simulink model "Controller_HIL"  (R2023b)
settings: Solver=FixedStepDiscrete  StartTime=0.0  StopTime=inf  FixedStep=ts_controller  RelTol=1e-3
InitFcn:
  | mbd_s32k_consistency_checks(bdroot(gcs));
undefined symbols (not defined in the file): Battery, BMS_Controller_State, Charging_State, currentFactor, CV_Gain, DiscIntNeverNeededParam, I_cc, LQFP, MaxCellVoltThrsld, noCurrent, Ns_Module, NumModules, OverCellVoltageLimit, SOCInit, SRE, ts_controller, ts_system, UnderCellVoltageLimit, voltThreshold
libraries: mbd_s32k1xx_ec_toolbox x20, mbd_bcc_ec_toolbox x16, etargetslib x11, simulink x5, sharedTrackingLibrary x2, hdlsllib x1
(part 1 of 2)
settings Model: DataDictionary=System.sldd  EnableAccessToBaseWorkspace=off  Creator=vasileios.amoiridis  LastModifiedBy=jatin.anand
settings DataIOCC: ExternalInput=off  InitialState=off  SaveOutput=off  SignalLogging=off  SaveTime=off
settings OptimizationCC: DefaultParameterBehavior=Inlined  DefaultUnderspecifiedDataType=single  EnhancedBackFolding=on  PassReuseOutputArgsAs=Individual arguments  ZeroExternalMemoryAtStartup=off  ZeroInternalMemoryAtStartup=off  OptimizeBlockOrder=speed  DifferentSizesBufferReuse=on  OptimizationCustomize=off  EfficientTunableParamExpr=on
settings DebuggingCC: InheritedTsInSrcMsg=none  SingleTaskRateTransMsg=error  ParameterTunabilityLossMsg=error  UnconnectedInputMsg=error  UnconnectedOutputMsg=error  UnconnectedLineMsg=error  UnknownTsInhSupMsg=error
settings HardwareCC: ProdBitPerPointer=32  ProdBitPerSizeT=32  ProdBitPerPtrDiffT=32  ProdLargestAtomicInteger=Long  ProdLargestAtomicFloat=Double  ProdWordSize=32  ProdHWDeviceType=ARM Compatible->ARM Cortex
settings SFSimCC: MATLABDynamicMemAlloc=off
settings RTWCC: Description=Model Based Design Toolbox S32K1xx Code Generation Target  SystemTargetFile=mbd_s32k.tlc  MakeCommand=mbd_s32k_make_rtw COPY_MDLREF_INCLUDES=0  TemplateMakefile=mbd_s32k.tmf
settings CodeAppCC: ForceParamTrailComments=on  IgnoreCustomStorageClasses=off  OperatorAnnotations=on  SimulinkDataObjDesc=on  SFDataObjDesc=on  InsertBlockDesc=on
settings STFCustomTargetCC: MultiwordLength=256  CombineOutputUpdateFcns=on  ERTCustomFileBanners=on  SupportContinuousTime=off  SupportNonInlinedSFcns=off  RemoveResetFunc=on  MATLABClassNameForMDSCustomization=Simulink.SoftwareTarget.ERTCustomization  SystemTargetFile=mbd_s32k.tlc
settings ERTTargetCC: TargetLangStandard=C99 (ISO)  ParMdlRefBuildCompliant=off  CompOptLevelCompliant=off  ConcurrentExecutionCompliant=off  ModelStepFunctionPrototypeControlCompliant=off  CPPClassGenCompliant=off  UseToolchainInfoCompliant=off  InlinedParameterPlacement=NonHierarchical  ERTSrcFileBannerTemplate=mbd_ert_code_template.cgt  ERTHdrFileBannerTemplate=mbd_ert_code_template.cgt  ERTDataSrcFileTemplate=mbd_ert_code_template.cgt  ERTDataHdrFileTemplate=mbd_ert_code_template.cgt  ERTCustomFileTemplate=example_file_process.tlc

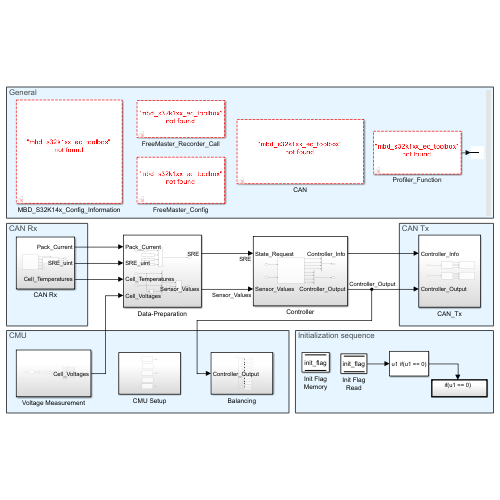
[thumbnail: Simulink's stored preview of the top-level diagram]
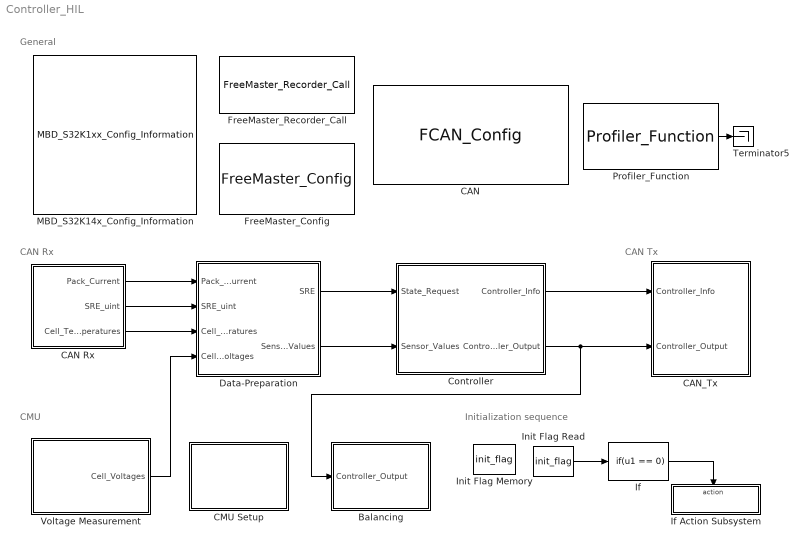
== system Controller_HIL ==
  note: CAN Tx
  note: CAN Rx
  note: CMU
  note: General
  note: Initialization sequence
  Balancing : Subsystem
  CAN : mbd_s32k1xx_ec_toolbox/Communication Blocks/CAN Blocks/FCAN_Config  Priority=1  can_instance=0  can_mode=Normal mode  can_max_num_mb=32  can_rx=PTE4: [CAN0_RX | CAN Rx channel]  can_tx=PTE5: [CAN0_TX | CAN Tx Channel]  show_adv_opts=on  can_clk_src=Peripheral clock  can_clk_freq=80 MHz  bitrate_to_time_seg=on  bitrate=1000  sample_point=80  real_bitrate=1000  real_sample_point=80  prop_delay=250  bus_length=1  tq=100.0  time_quanta=10  can_presdiv=8  can_propseg=6  can_pseg1=1  can_pseg2=2  can_rjw=1  cbt_bitrate=2000  cbt_sample_point=87.5  cbt_real_bitrate=2000  cbt_real_sample_point=80  cbt_tq=12.5  cbt_time_quanta=40  can_cbt_presdiv=1  can_cbt_propseg=29  can_cbt_pseg1=5  can_cbt_pseg2=5  can_cbt_rjw=5  can_fd_enable=off  can_payload=8  tdc_enable=off  tdc_offset=20  can_rxfifo_enable=on  can_num_id_filters=16  can_fifo_id_format=A  can_fifo_id_filter={{false,false,'0x401'},{false,false,'0x402'},{false,false,'0x403'},{false,false,'0x404'},{false,false,'0x405'},{false,false,'0x406'},{false,false,'0x407'},{false,false,'0x408'},{false,false,'0x409'},{false,false,'0x0'},{false,false,'0x0'},{false,false,'0x0'},{false,false,'0x0'},{false,false,'0x0'},{false,false,'0x0'},{false,false,'0x0'}}  can_pn_enable=off  can_wakeup_match=off  can_wakeup_timeout=off  can_timeout_en=off  can_match_timeout=1  can_multiple_matches_en=off  can_num_matches=1  can_idfilter_extendedid=off  can_idfilter_remoteframe=off  can_idfilter_type=Match exact  can_idfilter_id1=0  can_idfilter_id2=0  can_payloadfilter_enable=off  can_payloadfilter_dlclow=0  can_payloadfilter_dlchigh=0  can_payloadfilter_type=Match exact  can_payloadfilter_payload1_b0=0  can_payloadfilter_payload1_b1=0  can_payloadfilter_payload1_b2=0  can_payloadfilter_payload1_b3=0  can_payloadfilter_payload1_b4=0  can_payloadfilter_payload1_b5=0  can_payloadfilter_payload1_b6=0  can_payloadfilter_payload1_b7=0  can_payloadfilter_payload2_b0=0  can_payloadfilter_payload2_b1=0  can_payloadfilter_payload2_b2=0  can_payloadfilter_payload2_b3=0  can_payloadfilter_payload2_b4=0  can_payloadfilter_payload2_b5=0  can_payloadfilter_payload2_b6=0  can_payloadfilter_payload2_b7=0
  CAN Rx : Subsystem
  CAN_Tx : Subsystem
  CMU Setup : Subsystem
  Controller : Subsystem
  Data-Preparation : Subsystem
  FreeMaster_Config : mbd_s32k1xx_ec_toolbox/Utility Blocks/FreeMaster_Config  interface=LPUART1  baudrate=115200  rxd=PTC6: [LPUART1_RX | Receive]  txd=PTC7: [LPUART1_TX | Transmit]  mode=Short Interrupt  isr_prio=1  show_adv_opts=on  use_scope=on  max_scope_vars=8  use_recorder=on  max_rec_vars=8  rec_buff_size=512  rec_timebase=100 milliseconds  comm_buffer_size_auto=on  comm_buffer_size=255  comm_rqueue_size_default=on  comm_rqueue_size=32
  FreeMaster_Recorder_Call : mbd_s32k1xx_ec_toolbox/Utility Blocks/FreeMaster_Recorder_Call
  If : If  IfExpression=u1 == 0  ShowElse=off
  If Action Subsystem : Subsystem  TreatAsAtomicUnit=on
  Init Flag Memory : DataStoreMemory  DataStoreName=init_flag  ReadBeforeWriteMsg=warning  WriteAfterWriteMsg=warning  WriteAfterReadMsg=warning  ShowAdditionalParam=off  OutDataTypeStr=uint32
  Init Flag Read : DataStoreRead  DataStoreName=init_flag  IndexOptions=Index vector (dialog)  Indices=1  OutputSizes=1
  MBD_S32K14x_Config_Information : mbd_s32k1xx_ec_toolbox/MBD_S32K1xx_Config_Information  Priority=0  mbdt_ver=0  disp_str=|  config_params=[]  mcu_target_name=S32K144  mcu_target_package=100-LQFP  mcu_target_sram_size=48KB  mcu_system_clock_freq=80  mcu_xtal_freq=External 8  mcu_steptick_timer=LPIT Channel 0  mcu_steptick_prio=3  ds_import_enable=on  target_compiler=GCC  target_memory=FLASH  gcc_target_compile_opts=-mthumb -mfloat-abi=hard -mfpu=fpv4-sp-d16 -O1 -g -gstrict-dwarf  gcc_target_assemble_opts=-mthumb -mfloat-abi=hard -mfpu=fpv4-sp-d16 -g  gcc_target_link_opts=-mthumb -mfloat-abi=hard -mfpu=fpv4-sp-d16  gcc_target_default_lcf=on  gcc_target_user_lcf=S32K144_48_flash.ld  ghs_target_compile_opts=-cpu=cortexm4f -thumb -DARM_MATH_CM4 -fpu=vfpv4_d16 -fsingle -Ogeneral -Wundef -Wimplicit-int -Wshadow -Wtrigraphs --no_commons --gnu_asm -gnu99 -gdwarf-2 -G  ghs_target_assemble_opts=-cpu=cortexm4f -fpu=vfpv4_d16  ghs_target_link_opts=-cpu=cortexm4f -thumb -fpu=vfpv4_d16  ghs_target_default_lcf=off  ghs_target_user_lcf=S32K144_48_flash.ld  iar_target_compile_opts=--cpu=Cortex-M4F --thumb --fpu=VFPv4_sp -Ol -e --debug --dlib_config normal  iar_target_assemble_opts=--cpu Cortex-M4F --thumb --fpu VFPv4_sp  iar_target_link_opts=--no_exceptions --vfe --inline  iar_target_default_lcf=off  iar_target_user_lcf=S32K144_48_flash.icf  pil_download_enable=off  rbl_download_enable=on  rbl_start_delay=5000000  rbl_download_interface=OpenSDA  rbl_restart_request=off  rbl_com_port=Custom  rbl_com_port_custom=COM1  pil_download_rate=57600  pil_download_rate_custom=115200  pil_opensda_drive=Custom  pil_opensda_drive_custom=D  jtag_interface=OpenSDA Embedded Debug  jlink_default_path=on  jlink_user_path=C:\Program Files\SEGGER\JLink\  pil_uart_instance=1  pil_uart_rx=PTC6: [LPUART1_RX | Receive]  pil_uart_tx=PTC7: [LPUART1_TX | Transmit]  FTM_PWM_PcrCheckEnDis=on  FTM_Input_Edge_Inputs_PcrCheckEnDis=on  FTM_Dual_Edge_Inputs_PcrCheckEnDis=on  FTM_Quadrature_Inputs_PcrCheckEnDis=on  FTM_Hall_Sensor_Inputs_PcrCheckEnDis=on  LPTMR_PcrCheckEnDis=on  PIT_PcrCheckEnDis=on  RTC_PcrCheckEnDis=on  FlexCAN_PcrCheckEnDis=on  LIN_PcrCheckEnDis=on  FlexIO_PcrCheckEnDis=on  LPI2C_PcrCheckEnDis=on  LPSPI_PcrCheckEnDis=on  LPUART_PcrCheckEnDis=on  CMP_PcrCheckEnDis=on  GPIO_OutputPcrCheckEnDis=on  GPIO_InputPcrCheckEnDis=on  SBC_PcrCheckEnDis=on  BMS_PcrCheckEnDis=on  AMMCLIB_PcrCheckEnDis=on  FM_PcrCheckEnDis=on  Profile_PcrCheckEnDis=on  ConfigParams_PcrCheckEnDis=on  ModelRef_PcrCheckEnDis=on  PDB0_PcrCheckEnDis=on  CSEc_PcrCheckEnDis=on  eDMA_PcrCheckEnDis=on  FLASH_PcrCheckEnDis=on  ADC_PcrCheckEnDis=on  WDOG_PcrCheckEnDis=on
      | Target : S32K144-64KB_SRAM
      | Package : 100-pin
      | System clock : 80 MHz
      | XTAL clock : External 8 MHz
      | Compiler : GCC
      | Target Type : FLASH
      | Download Code after build : (OpenSDA: E)
      | Step Tick Interrupt Priority : 15
  Profiler_Function : mbd_s32k1xx_ec_toolbox/Utility Blocks/Profiler_Function  profile_indx=0
      settings: showOut=on
  Terminator5 : Terminator
  Voltage Measurement : Subsystem
  wires:
  Controller/2(Controller_Output) -> Balancing/1(Controller_Output), CAN_Tx/2(Controller_Output)
  Profiler_Function/1 -> Terminator5/1
  Data-Preparation/2(Sensor_Values) -> Controller/2(Sensor_Values)
  Controller/1(Controller_Info) -> CAN_Tx/1(Controller_Info)
  If/1 -> If Action Subsystem/Action
  Data-Preparation/1(SRE) -> Controller/1(State_Request)
  Init Flag Read/1 -> If/1
  CAN Rx/1(Pack_Current) -> Data-Preparation/1(Pack_Current)
  CAN Rx/2(SRE_uint) -> Data-Preparation/2(SRE_uint)
  CAN Rx/3(Cell_Temperatures) -> Data-Preparation/3(Cell_Temperatures)
  Voltage Measurement/1(Cell_Voltages) -> Data-Preparation/4(Cell_Voltages)

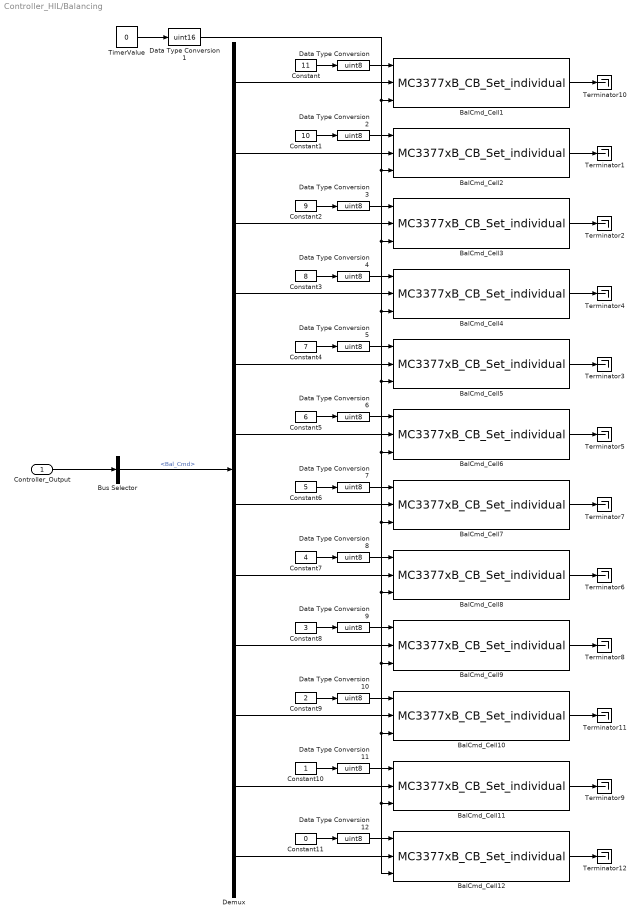
== system Controller_HIL/Balancing ==
  Controller_Output : Inport
  BalCmd_Cell{1..12} (12 alike) : mbd_bcc_ec_toolbox/BMS/MC3377xB_CB_Set_individual  bccInstance=0  bccCID=1
  Bus Selector : BusSelector  OutputSignals=Bal_Cmd
  Constant : Constant  Value=11  SampleTime=-1
  Constant1 : Constant  Value=10  SampleTime=-1
  Constant10 : Constant  SampleTime=-1
  Constant11 : Constant  Value=0  SampleTime=-1
  Constant2 : Constant  Value=9  SampleTime=-1
  Constant3 : Constant  Value=8  SampleTime=-1
  Constant4 : Constant  Value=7  SampleTime=-1
  Constant5 : Constant  Value=6  SampleTime=-1
  Constant6 : Constant  Value=5  SampleTime=-1
  Constant7 : Constant  Value=4  SampleTime=-1
  Constant8 : Constant  Value=3  SampleTime=-1
  Constant9 : Constant  Value=2  SampleTime=-1
  Data Type Conversion{,2..12} (12 alike) : DataTypeConversion  OutDataTypeStr=uint8  SaturateOnIntegerOverflow=off  RndMeth=Floor
  Data Type Conversion1 : DataTypeConversion  OutDataTypeStr=uint16  SaturateOnIntegerOverflow=off  RndMeth=Floor
  Demux : Demux  Outputs=12
  Terminator{1..12} (12 alike) : Terminator
  TimerValue : Constant  Value=0  SampleTime=-1
  wires:
  Demux/12 -> BalCmd_Cell12/2
  Demux/3 -> BalCmd_Cell3/2
  BalCmd_Cell6/1 -> Terminator5/1
  Constant10/1 -> Data Type Conversion11/1
  Demux/10 -> BalCmd_Cell10/2
  BalCmd_Cell10/1 -> Terminator11/1
  Data Type Conversion6/1 -> BalCmd_Cell6/1
  Demux/1 -> BalCmd_Cell1/2
  Demux/5 -> BalCmd_Cell5/2
  Constant8/1 -> Data Type Conversion9/1
  Constant11/1 -> Data Type Conversion12/1
  TimerValue/1 -> Data Type Conversion1/1
  Constant6/1 -> Data Type Conversion7/1
  Data Type Conversion8/1 -> BalCmd_Cell8/1
  Data Type Conversion9/1 -> BalCmd_Cell9/1
  Data Type Conversion5/1 -> BalCmd_Cell5/1
  Constant9/1 -> Data Type Conversion10/1
  Bus Selector/1 -> Demux/1  "<Bal_Cmd>"
  Demux/11 -> BalCmd_Cell11/2
  Data Type Conversion1/1 -> BalCmd_Cell5/3, BalCmd_Cell11/3, BalCmd_Cell12/3, BalCmd_Cell10/3, BalCmd_Cell9/3, BalCmd_Cell8/3, BalCmd_Cell7/3, BalCmd_Cell6/3, BalCmd_Cell4/3, BalCmd_Cell3/3, BalCmd_Cell2/3, BalCmd_Cell1/3
  Demux/9 -> BalCmd_Cell9/2
  BalCmd_Cell7/1 -> Terminator7/1
  Demux/8 -> BalCmd_Cell8/2
  Demux/2 -> BalCmd_Cell2/2
  Demux/7 -> BalCmd_Cell7/2
  Data Type Conversion11/1 -> BalCmd_Cell11/1
  Constant7/1 -> Data Type Conversion8/1
  Constant/1 -> Data Type Conversion/1
  BalCmd_Cell12/1 -> Terminator12/1
  Data Type Conversion7/1 -> BalCmd_Cell7/1
  Data Type Conversion10/1 -> BalCmd_Cell10/1
  BalCmd_Cell5/1 -> Terminator3/1
  BalCmd_Cell8/1 -> Terminator6/1
  Demux/4 -> BalCmd_Cell4/2
  Demux/6 -> BalCmd_Cell6/2
  BalCmd_Cell3/1 -> Terminator2/1
  Controller_Output/1 -> Bus Selector/1
  Data Type Conversion12/1 -> BalCmd_Cell12/1
  Constant3/1 -> Data Type Conversion4/1
  Constant1/1 -> Data Type Conversion2/1
  BalCmd_Cell1/1 -> Terminator10/1
  BalCmd_Cell2/1 -> Terminator1/1
  Constant2/1 -> Data Type Conversion3/1
  Data Type Conversion/1 -> BalCmd_Cell1/1
  BalCmd_Cell4/1 -> Terminator4/1
  BalCmd_Cell9/1 -> Terminator8/1
  Constant5/1 -> Data Type Conversion6/1
  Data Type Conversion3/1 -> BalCmd_Cell3/1
  Data Type Conversion2/1 -> BalCmd_Cell2/1
  Data Type Conversion4/1 -> BalCmd_Cell4/1
  BalCmd_Cell11/1 -> Terminator9/1
  Constant4/1 -> Data Type Conversion5/1

== system Controller_HIL/CAN Rx ==
  FCAN_Rx_FIFO_Complete_Isr : mbd_s32k1xx_ec_toolbox/Communication Blocks/CAN Blocks/FCAN_Isr  can_instance=0  can_event=Rx FIFO Complete
  RX_FIFO_Complete_Event : Subsystem
  Terminator : Terminator
  Terminator1 : Terminator
  Pack_Current : Outport
  SRE_uint : Outport  Port=2
  Cell_Temperatures : Outport  Port=3
  wires:
  FCAN_Rx_FIFO_Complete_Isr/4 -> Terminator/1
  FCAN_Rx_FIFO_Complete_Isr/5 -> Terminator1/1
  FCAN_Rx_FIFO_Complete_Isr/2 -> RX_FIFO_Complete_Event/1(ID)
  FCAN_Rx_FIFO_Complete_Isr/3 -> RX_FIFO_Complete_Event/2(Data)
  FCAN_Rx_FIFO_Complete_Isr/1 -> RX_FIFO_Complete_Event/Trigger
  RX_FIFO_Complete_Event/1(Pack_Current) -> Pack_Current/1
  RX_FIFO_Complete_Event/2(SRE_uint) -> SRE_uint/1
  RX_FIFO_Complete_Event/3(Cell_Temperatures) -> Cell_Temperatures/1

== system Controller_HIL/CAN_Tx ==
  Controller_Info : Inport
  Controller_Output : Inport  Port=2
  CAN_Data : Subsystem
  CAN_Data_HIL : Subsystem
  TX_Complete_HIL : Subsystem  TreatAsAtomicUnit=on
  Tx_Complete : Subsystem  TreatAsAtomicUnit=on
  wires:
  CAN_Data/4(Length_0x202) -> Tx_Complete/4(Length_0x202)
  CAN_Data/3(Data_0x202) -> Tx_Complete/3(Data_0x202)
  CAN_Data/1(Data_0x201) -> Tx_Complete/1(Data_0x201)
  CAN_Data/2(Length_0x201) -> Tx_Complete/2(Length_0x201)
  CAN_Data_HIL/1(Data_0x501) -> TX_Complete_HIL/1(Data_0x501)
  CAN_Data_HIL/2(Length_0x501) -> TX_Complete_HIL/2(Length_0x501)
  CAN_Data_HIL/4(Length_0x502) -> TX_Complete_HIL/4(Length_0x502)
  CAN_Data_HIL/3(Data_0x502) -> TX_Complete_HIL/3(Data_0x502)
  Controller_Info/1 -> CAN_Data_HIL/1(Controller_Info)
  Controller_Output/1 -> CAN_Data/1(Controller_Output)

== system Controller_HIL/CMU Setup ==
  "LPSPI_RX " : mbd_s32k1xx_ec_toolbox/Communication Blocks/SPI Blocks/LPSPI_Config   InstanceNumber=0  Role=Slave  BaudRate=1000000  ShowAdvanced=on  sin=PTB3: [LPSPI0_SIN | LPSPI Serial Data Input]  sout=None  sck=PTB2: [LPSPI0_SCK | LPSPI Serial Clock I/O]  pcs0=None  pcs1=PTB5: [LPSPI0_PCS1 | Peripheral Chip Select 1]  pcs2=None  pcs3=None  CPHA=1  CPOL=0  BitOrder=MSB first  TransferSize=40  WhichPCS=1  PCSPol=ActiveLow  ContinuousTransfer=off
  LPSPI_TX : mbd_s32k1xx_ec_toolbox/Communication Blocks/SPI Blocks/LPSPI_Config   InstanceNumber=1  Role=Master  BaudRate=2000000  ShowAdvanced=on  sin=None  sout=PTB16: [LPSPI1_SOUT | LPSPI Serial Data Output]  sck=PTB14: [LPSPI1_SCK | LPSPI Serial Clock I/O]  pcs0=PTD3: [LPSPI1_PCS0 | Peripheral Chip Select 0]  pcs1=PTA6: [LPSPI1_PCS1 | Peripheral Chip Select 1]  pcs2=None  pcs3=None  CPHA=1  CPOL=0  BitOrder=MSB first  TransferSize=40  WhichPCS=1  PCSPol=ActiveLow  ContinuousTransfer=off
  MC3377xB_CB_Disable_Enable : mbd_bcc_ec_toolbox/BMS/MC3377xB_CB_Disable_Enable  bccInstance=0  bccCID=1  bccAction=Enable
  MC3377xB_Config : mbd_bcc_ec_toolbox/BMS/MC3377xB_Config  Priority=1  bccInstance=0  bccMode=TPL  bccTPLDevNr=1  bccSpiDev=MC33771B  bccSpiCell=3  bccTPLDev1=MC33771B  bccTPLCell1=14  bccTPLDev2=MC33771B  bccTPLCell2=3  bccTPLDev3=MC33771B  bccTPLCell3=3  bccTPLDev4=MC33771B  bccTPLCell4=3  bccTPLDev5=MC33771B  bccTPLCell5=3  bccTPLDev6=MC33771B  bccTPLCell6=3  bccTPLDev7=MC33771B  bccTPLCell7=3  bccTPLDev8=MC33771B  bccTPLCell8=3  bccTPLDev9=MC33771B  bccTPLCell9=3  bccTPLDev10=MC33771B  bccTPLCell10=3  bccTPLDev11=MC33771B  bccTPLCell11=3  bccTPLDev12=MC33771B  bccTPLCell12=3  bccTPLDev13=MC33771B  bccTPLCell13=3  bccTPLDev14=MC33771B  bccTPLCell14=3  bccTPLDev15=MC33771B  bccTPLCell15=3  bccSpiMaster=1  bccSPIMasterCSCustom=off  bccSPIMasterPCS=LPSPI_PCS1  bccSPIMasterPCSGPIO=PTA0: [PTA0 | Port A I/O]  bccSpiSlave=0  bccSPISlavePCS=LPSPI_PCS1  bccSPI_RESET_ALT0=PTA0: [PTA0 | Port A I/O]  bccTPL_ENABLE=PTB0: [PTB0 | Port B I/O]  bccTPL_INTB=PTB1: [PTB1 | Port B I/O]  bccNTCBeta=3900  bccNTCRes=6800  bccNTCRefR=10000  bccNTCRefT=25  bccShunt=10000
  MC3377xB_Start_Conversion : mbd_bcc_ec_toolbox/BMS/MC3377xB_Start_Conversion  Priority=100  bccInstance=0  bccCID=1  bccCIDGlobal=on  bccADCCFG=0
  Terminator : Terminator
  Terminator1 : Terminator
  Terminator2 : Terminator
  wires:
  MC3377xB_CB_Disable_Enable/1 -> Terminator/1
  MC3377xB_Config/1 -> Terminator2/1
  MC3377xB_Start_Conversion/1 -> Terminator1/1

== system Controller_HIL/Controller ==
  State_Request : Inport  OutDataTypeStr=Enum: SRE  PortDimensions=1
  Sensor_Values : Inport  Port=2  OutDataTypeStr=Bus: Sensor_Values  BusOutputAsStruct=on
  Bus Creator : BusCreator  Inputs=4  OutDataTypeStr=Bus: Controller_Info
  Bus Creator1 : BusCreator  Inputs=4  OutDataTypeStr=Bus: Controller_Output  NonVirtualBus=on
      settings: InheritFromInputs=off
  Controller : Subsystem
  Controller_Info : Outport
  Controller_Output : Outport  Port=2  OutDataTypeStr=Bus: Controller_Output  VectorParamsAs1DForOutWhenUnconnected=off  BusOutputAsStruct=on
  wires:
  Sensor_Values/1 -> Controller/1(Sensor_Values)
  Controller/8(Bal_Cmd) -> Bus Creator1/4
  Controller/5(Discharge_Current_Limit) -> Bus Creator1/1
  Controller/6(Charge_Current_Limit) -> Bus Creator1/2
  Bus Creator1/1 -> Controller_Output/1  "Controller_Output"
  Bus Creator/1 -> Controller_Info/1  "Controller_Info"
  State_Request/1 -> Controller/2(State_Request)
  Controller/4(SOC) -> Bus Creator/4
  Controller/3(BMS_Controller_State) -> Bus Creator/3
  Controller/2(Charging_State) -> Bus Creator/2
  Controller/7(Charge_Current_Req) -> Bus Creator1/3
  Controller/1(Faults) -> Bus Creator/1

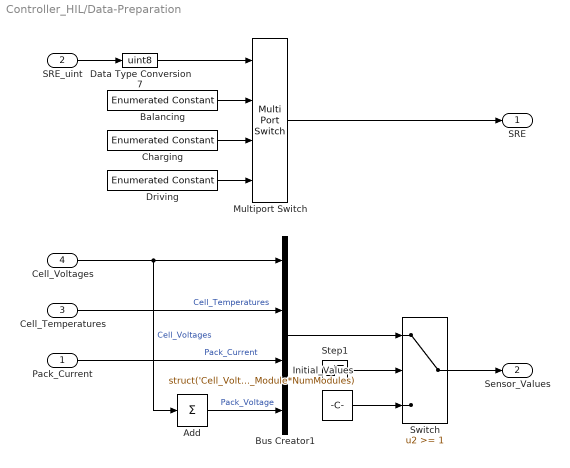
== system Controller_HIL/Data-Preparation ==
  Pack_Current : Inport
  SRE_uint : Inport  Port=2
  Cell_Temperatures : Inport  Port=3
  Cell_Voltages : Inport  Port=4
  Add : Sum  Inputs=+
  Balancing : simulink/Sources/Enumerated Constant  OutDataTypeStr=Enum: SRE  Value=SRE.Standby  SampleTime=-1
  Bus Creator1 : BusCreator  Inputs=4  OutDataTypeStr=Bus: Sensor_Values  NonVirtualBus=on
  Charging : simulink/Sources/Enumerated Constant  OutDataTypeStr=Enum: SRE  Value=SRE.Driving  SampleTime=-1
  Data Type Conversion7 : DataTypeConversion  OutDataTypeStr=uint8  SaturateOnIntegerOverflow=off  RndMeth=Floor
  Driving : simulink/Sources/Enumerated Constant  OutDataTypeStr=Enum: SRE  Value=SRE.Charging  SampleTime=-1
  Initial_Values : Constant  Value=struct('Cell_Voltages',3.6*ones(1, Ns_Module*NumModules),'Cell_Temperatures',293.15*ones(1,Ns_Module*NumModules),'Pack_Current',0,'Pack_Voltage',3.6*Ns_Module*NumModules)  OutDataTypeStr=Bus: Sensor_Values  SampleTime=-1
  Multiport Switch : MultiPortSwitch  DataPortOrder=Zero-based contiguous  zeroidx=on  SaturateOnIntegerOverflow=off  InputSameDT=off
  Step1 : Step
  Switch : Switch  Threshold=1  SaturateOnIntegerOverflow=off  InputSameDT=off
  SRE : Outport
  Sensor_Values : Outport  Port=2
  wires:
  Bus Creator1/1 -> Switch/1
  Step1/1 -> Switch/2
  Pack_Current/1 -> Bus Creator1/3  "Pack_Current"
  Cell_Temperatures/1 -> Bus Creator1/2  "Cell_Temperatures"
  Multiport Switch/1 -> SRE/1
  Switch/1 -> Sensor_Values/1
  Driving/1 -> Multiport Switch/4
  Charging/1 -> Multiport Switch/3
  Balancing/1 -> Multiport Switch/2
  Data Type Conversion7/1 -> Multiport Switch/1
  Initial_Values/1 -> Switch/3
  Add/1 -> Bus Creator1/4  "Pack_Voltage"
  SRE_uint/1 -> Data Type Conversion7/1
  Cell_Voltages/1 -> Bus Creator1/1, Add/1  "Cell_Voltages"

== system Controller_HIL/If Action Subsystem ==
  Action Port : ActionPort  ActionPortLabel=if(u1 == 0)
  Constant : Constant  OutDataTypeStr=uint32  SampleTime=-1
  FCAN_Receive_FIFO : mbd_s32k1xx_ec_toolbox/Communication Blocks/CAN Blocks/FCAN_Receive  can_instance=0  can_mode=Non-blocking  can_timeout_ms=0  can_mb_idx=0  can_mb_init=Once  show_id_input=off  can_extended_id=off  can_is_remote=off  can_id=0x7FF  can_msg_mask=0  show_adv_opts=on  can_use_rxfifo=on  can_fd_enable=off
  Init Flag Write : DataStoreWrite  DataStoreName=init_flag  IndexOptions=Index vector (dialog)  Indices=1  OutputSizes=1
  wires:
  Constant/1 -> Init Flag Write/1

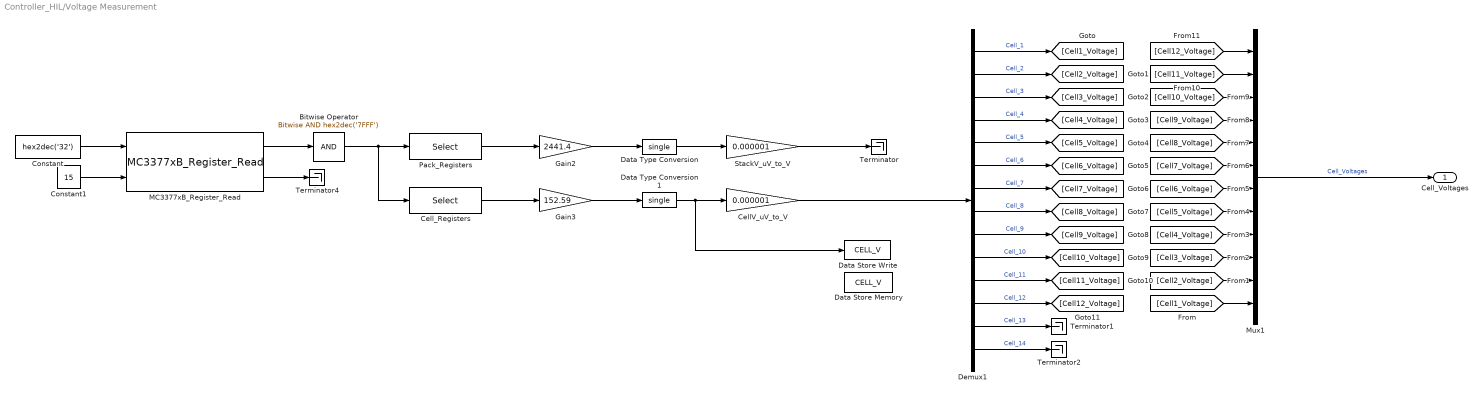
== system Controller_HIL/Voltage Measurement ==
  Bitwise Operator : simulink/Logic and Bit Operations/Bitwise Operator  logicop=AND  UseBitMask=on  BitMask=hex2dec('7FFF')  BitMaskRealWorld=Stored Integer
  CellV_uV_to_V : Gain  Gain=0.000001
  Cell_Registers : Selector  InputPortWidth=15  IndexOptions=Index vector (dialog)  Indices=[15 14 13 12 11 10 9 8 7 6 5 4 3 2]  OutputSizes=1
  Constant : Constant  Value=hex2dec('32')  OutDataTypeStr=Inherit: Inherit via back propagation  SampleTime=-1
  Constant1 : Constant  Value=15  OutDataTypeStr=Inherit: Inherit via back propagation  SampleTime=-1
  Data Store Memory : DataStoreMemory  DataStoreName=CELL_V  WriteAfterWriteMsg=warning  InitialValue=zeros(14,1)  ShowAdditionalParam=off
  Data Store Write : DataStoreWrite  DataStoreName=CELL_V  IndexOptions=Index vector (dialog)  Indices=1  OutputSizes=1
  Data Type Conversion : DataTypeConversion  OutDataTypeStr=single  SaturateOnIntegerOverflow=off  RndMeth=Floor
  Data Type Conversion1 : DataTypeConversion  OutDataTypeStr=single  SaturateOnIntegerOverflow=off  RndMeth=Floor
  Demux1 : Demux  Outputs=14
  Gain2 : Gain  Gain=2441.4
  Gain3 : Gain  Gain=152.59
  MC3377xB_Register_Read : mbd_bcc_ec_toolbox/BMS/MC3377xB_Register_Read  bccInstance=0  bccCID=1
  Mux1 : Mux  Inputs=12
  Pack_Registers : Selector  InputPortWidth=15  IndexOptions=Index vector (dialog)  Indices=[1]  OutputSizes=1
  StackV_uV_to_V : Gain  Gain=0.000001
  Terminator{,1..2,4} (4 alike) : Terminator
  Cell_Voltages : Outport
  wires:
  [Cell7_Voltage] -> Mux1/6
  [Cell9_Voltage] -> Mux1/4
  Mux1/1 -> Cell_Voltages/1  "Cell_Voltages"
  [Cell11_Voltage] -> Mux1/2
  [Cell4_Voltage] -> Mux1/9
  Pack_Registers/1 -> Gain2/1
  [Cell5_Voltage] -> Mux1/8
  Demux1/12 -> [Cell12_Voltage]  "Cell_12"
  [Cell10_Voltage] -> Mux1/3
  CellV_uV_to_V/1 -> Demux1/1
  Demux1/13 -> Terminator1/1  "Cell_13"
  Demux1/10 -> [Cell10_Voltage]  "Cell_10"
  Demux1/2 -> [Cell2_Voltage]  "Cell_2"
  [Cell3_Voltage] -> Mux1/10
  [Cell2_Voltage] -> Mux1/11
  [Cell1_Voltage] -> Mux1/12
  Demux1/14 -> Terminator2/1  "Cell_14"
  Demux1/7 -> [Cell7_Voltage]  "Cell_7"
  Constant1/1 -> MC3377xB_Register_Read/2
  [Cell12_Voltage] -> Mux1/1
  Demux1/3 -> [Cell3_Voltage]  "Cell_3"
  [Cell6_Voltage] -> Mux1/7
  Data Type Conversion1/1 -> Data Store Write/1, CellV_uV_to_V/1
  Demux1/11 -> [Cell11_Voltage]  "Cell_11"
  Demux1/9 -> [Cell9_Voltage]  "Cell_9"
  Gain2/1 -> Data Type Conversion/1
  Demux1/1 -> [Cell1_Voltage]  "Cell_1"
  Data Type Conversion/1 -> StackV_uV_to_V/1
  Bitwise Operator/1 -> Cell_Registers/1, Pack_Registers/1
  Cell_Registers/1 -> Gain3/1
  [Cell8_Voltage] -> Mux1/5
  Demux1/6 -> [Cell6_Voltage]  "Cell_6"
  Gain3/1 -> Data Type Conversion1/1
  Demux1/5 -> [Cell5_Voltage]  "Cell_5"
  MC3377xB_Register_Read/1 -> Bitwise Operator/1
  Demux1/8 -> [Cell8_Voltage]  "Cell_8"
  Demux1/4 -> [Cell4_Voltage]  "Cell_4"
  StackV_uV_to_V/1 -> Terminator/1
  MC3377xB_Register_Read/2 -> Terminator4/1
  Constant/1 -> MC3377xB_Register_Read/1

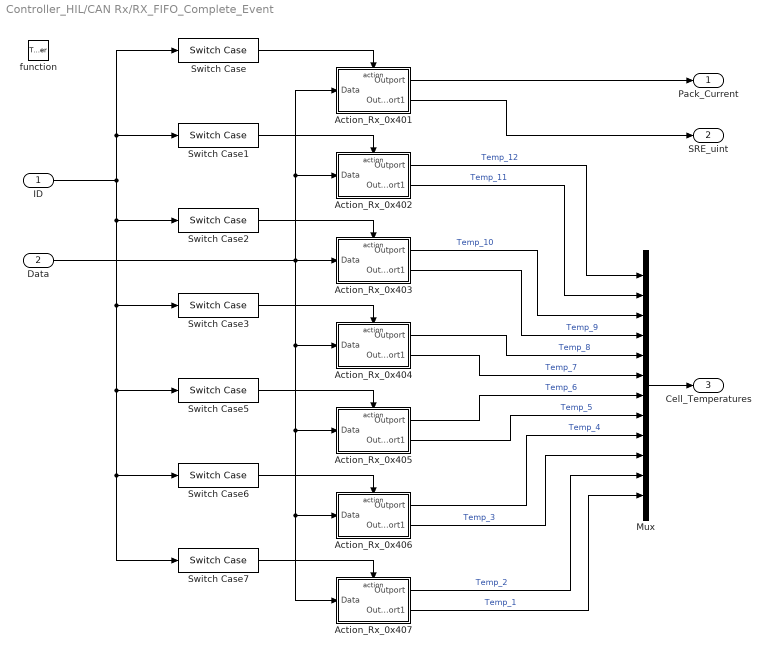
== system Controller_HIL/CAN Rx/RX_FIFO_Complete_Event ==
  ID : Inport
  Data : Inport  Port=2
  function : TriggerPort  TriggerType=function-call  VariantControl=Variant
  Action_Rx_0x401 : Subsystem  TreatAsAtomicUnit=on
  Action_Rx_0x402 : Subsystem  TreatAsAtomicUnit=on
  Action_Rx_0x403 : Subsystem  TreatAsAtomicUnit=on
  Action_Rx_0x404 : Subsystem  TreatAsAtomicUnit=on
  Action_Rx_0x405 : Subsystem  TreatAsAtomicUnit=on
  Action_Rx_0x406 : Subsystem  TreatAsAtomicUnit=on
  Action_Rx_0x407 : Subsystem  TreatAsAtomicUnit=on
  Mux : Mux  Inputs=12
  Switch Case : SwitchCase  CaseConditions={hex2dec('401')}  ShowDefaultCase=off
  Switch Case1 : SwitchCase  CaseConditions={hex2dec('402')}  ShowDefaultCase=off
  Switch Case2 : SwitchCase  CaseConditions={hex2dec('403')}  ShowDefaultCase=off
  Switch Case3 : SwitchCase  CaseConditions={hex2dec('404')}  ShowDefaultCase=off
  Switch Case5 : SwitchCase  CaseConditions={hex2dec('405')}  ShowDefaultCase=off
  Switch Case6 : SwitchCase  CaseConditions={hex2dec('406')}  ShowDefaultCase=off
  Switch Case7 : SwitchCase  CaseConditions={hex2dec('407')}  ShowDefaultCase=off
  Pack_Current : Outport
  SRE_uint : Outport  Port=2
  Cell_Temperatures : Outport  Port=3
  wires:
  Data/1 -> Action_Rx_0x405/1(Data), Action_Rx_0x406/1(Data), Action_Rx_0x407/1(Data), Action_Rx_0x404/1(Data), Action_Rx_0x403/1(Data), Action_Rx_0x402/1(Data), Action_Rx_0x401/1(Data)
  ID/1 -> Switch Case3/1, Switch Case5/1, Switch Case6/1, Switch Case7/1, Switch Case2/1, Switch Case1/1, Switch Case/1
  Action_Rx_0x406/1(Outport) -> Mux/9  "Temp_4"
  Action_Rx_0x407/1(Outport) -> Mux/11  "Temp_2"
  Switch Case/1 -> Action_Rx_0x401/Action
  Action_Rx_0x405/2(Outport1) -> Mux/8  "Temp_5"
  Action_Rx_0x405/1(Outport) -> Mux/7  "Temp_6"
  Action_Rx_0x406/2(Outport1) -> Mux/10  "Temp_3"
  Switch Case3/1 -> Action_Rx_0x404/Action
  Action_Rx_0x402/1(Outport) -> Mux/1  "Temp_12"
  Switch Case5/1 -> Action_Rx_0x405/Action
  Switch Case7/1 -> Action_Rx_0x407/Action
  Action_Rx_0x404/2(Outport1) -> Mux/6  "Temp_7"
  Switch Case1/1 -> Action_Rx_0x402/Action
  Mux/1 -> Cell_Temperatures/1
  Switch Case6/1 -> Action_Rx_0x406/Action
  Switch Case2/1 -> Action_Rx_0x403/Action
  Action_Rx_0x407/2(Outport1) -> Mux/12  "Temp_1"
  Action_Rx_0x403/2(Outport1) -> Mux/4  "Temp_9"
  Action_Rx_0x401/2(Outport1) -> SRE_uint/1
  Action_Rx_0x403/1(Outport) -> Mux/3  "Temp_10"
  Action_Rx_0x402/2(Outport1) -> Mux/2  "Temp_11"
  Action_Rx_0x401/1(Outport) -> Pack_Current/1
  Action_Rx_0x404/1(Outport) -> Mux/5  "Temp_8"

== system Controller_HIL/CAN_Tx/CAN_Data ==
  Controller_Output : Inport
  Bus Selector : BusSelector  OutputSignals=Discharge_Current_Limit,Charge_Current_Limit,Charge_Current_Req
  Byte Pack : etargetslib/Byte Pack  datatypes={'single','single'}  byteAlign=1
  Byte Pack1 : etargetslib/Byte Pack  datatypes={'single'}  byteAlign=1
  Probe : Probe  ProbeSampleTime=off  ProbeComplexSignal=off  ProbeWidthDataType=Same as input
  Probe1 : Probe  ProbeSampleTime=off  ProbeComplexSignal=off  ProbeWidthDataType=Same as input
  Data_0x201 : Outport
  Length_0x201 : Outport  Port=2
  Data_0x202 : Outport  Port=3
  Length_0x202 : Outport  Port=4
  wires:
  Bus Selector/3 -> Byte Pack1/1  "<Charge_Current_Req>"
  Controller_Output/1 -> Bus Selector/1
  Probe/1 -> Length_0x201/1
  Byte Pack/1 -> Probe/1, Data_0x201/1
  Byte Pack1/1 -> Probe1/1, Data_0x202/1
  Probe1/1 -> Length_0x202/1
  Bus Selector/1 -> Byte Pack/1  "<Discharge_Current_Limit>"
  Bus Selector/2 -> Byte Pack/2  "<Charge_Current_Limit>"

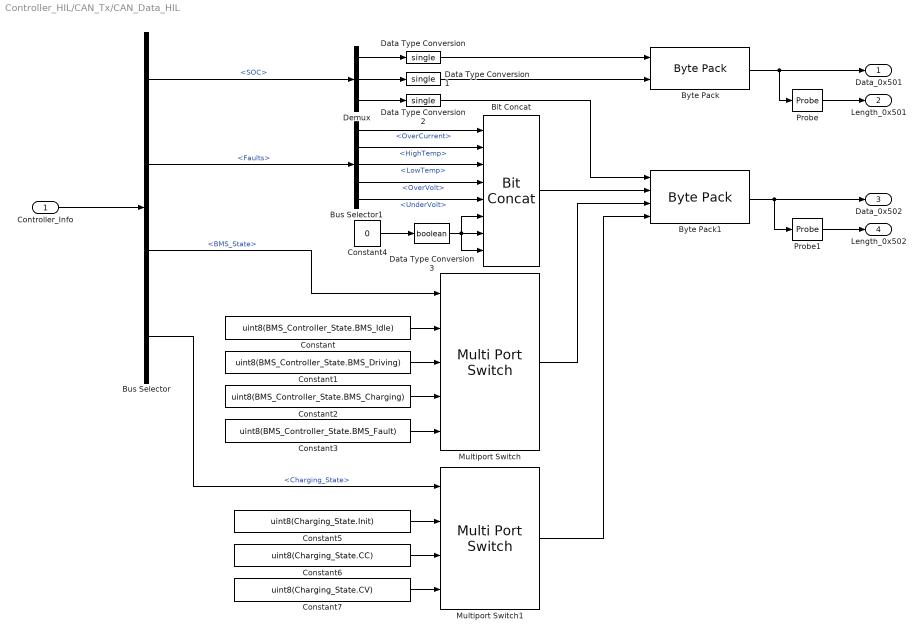
== system Controller_HIL/CAN_Tx/CAN_Data_HIL ==
  Controller_Info : Inport
  Bit Concat : hdlsllib/Logic and Bit Operations/Bit Concat  numInputs=8
  Bus Selector : BusSelector  OutputSignals=SOC,Faults,BMS_State,Charging_State
  Bus Selector1 : BusSelector  OutputSignals=OverCurrent,HighTemp,LowTemp,OverVolt,UnderVolt
  Byte Pack : etargetslib/Byte Pack  datatypes={'single','single'}  byteAlign=1
  Byte Pack1 : etargetslib/Byte Pack  datatypes={'single','uint8','uint8','uint8'}  byteAlign=1
  Constant : Constant  Value=uint8(BMS_Controller_State.BMS_Idle)  SampleTime=-1
  Constant1 : Constant  Value=uint8(BMS_Controller_State.BMS_Driving)  SampleTime=-1
  Constant2 : Constant  Value=uint8(BMS_Controller_State.BMS_Charging)  SampleTime=-1
  Constant3 : Constant  Value=uint8(BMS_Controller_State.BMS_Fault)  SampleTime=-1
  Constant4 : Constant  Value=0  SampleTime=-1
  Constant5 : Constant  Value=uint8(Charging_State.Init)  SampleTime=-1
  Constant6 : Constant  Value=uint8(Charging_State.CC)  SampleTime=-1
  Constant7 : Constant  Value=uint8(Charging_State.CV)  SampleTime=-1
  Data Type Conversion : DataTypeConversion  OutDataTypeStr=single  SaturateOnIntegerOverflow=off  RndMeth=Floor
  Data Type Conversion1 : DataTypeConversion  OutDataTypeStr=single  SaturateOnIntegerOverflow=off  RndMeth=Floor
  Data Type Conversion2 : DataTypeConversion  OutDataTypeStr=single  SaturateOnIntegerOverflow=off  RndMeth=Floor
  Data Type Conversion3 : DataTypeConversion  OutDataTypeStr=boolean  SaturateOnIntegerOverflow=off  RndMeth=Floor
  Demux : Demux  Outputs=3
  Multiport Switch : MultiPortSwitch  DataPortOrder=Specify indices  DataPortIndices={BMS_Controller_State.BMS_Idle, BMS_Controller_State.BMS_Driving, BMS_Controller_State.BMS_Charging, BMS_Controller_State.BMS_Fault}  OutDataTypeStr=uint8  SaturateOnIntegerOverflow=off  InputSameDT=off
  Multiport Switch1 : MultiPortSwitch  DataPortOrder=Specify indices  DataPortIndices={Charging_State.Init, Charging_State.CC, Charging_State.CV}  OutDataTypeStr=uint8  SaturateOnIntegerOverflow=off  InputSameDT=off
  Probe : Probe  ProbeSampleTime=off  ProbeComplexSignal=off  ProbeWidthDataType=Same as input
  Probe1 : Probe  ProbeSampleTime=off  ProbeComplexSignal=off  ProbeWidthDataType=Same as input
  Data_0x501 : Outport
  Length_0x501 : Outport  Port=2
  Data_0x502 : Outport  Port=3
  Length_0x502 : Outport  Port=4
  wires:
  Controller_Info/1 -> Bus Selector/1
  Probe/1 -> Length_0x501/1
  Byte Pack/1 -> Probe/1, Data_0x501/1
  Byte Pack1/1 -> Data_0x502/1, Probe1/1
  Probe1/1 -> Length_0x502/1
  Constant/1 -> Multiport Switch/2
  Constant1/1 -> Multiport Switch/3
  Constant2/1 -> Multiport Switch/4
  Constant3/1 -> Multiport Switch/5
  Demux/1 -> Data Type Conversion/1
  Demux/2 -> Data Type Conversion1/1
  Data Type Conversion/1 -> Byte Pack/1
  Data Type Conversion1/1 -> Byte Pack/2
  Demux/3 -> Data Type Conversion2/1
  Bit Concat/1 -> Byte Pack1/2
  Multiport Switch/1 -> Byte Pack1/3
  Data Type Conversion2/1 -> Byte Pack1/1
  Bus Selector/1 -> Demux/1  "<SOC>"
  Bus Selector/2 -> Bus Selector1/1  "<Faults>"
  Bus Selector/3 -> Multiport Switch/1  "<BMS_State>"
  Bus Selector1/1 -> Bit Concat/1  "<OverCurrent>"
  Bus Selector1/2 -> Bit Concat/2  "<HighTemp>"
  Bus Selector1/3 -> Bit Concat/3  "<LowTemp>"
  Bus Selector1/4 -> Bit Concat/4  "<OverVolt>"
  Bus Selector1/5 -> Bit Concat/5  "<UnderVolt>"
  Constant4/1 -> Data Type Conversion3/1
  Data Type Conversion3/1 -> Bit Concat/8, Bit Concat/6, Bit Concat/7
  Constant5/1 -> Multiport Switch1/2
  Constant7/1 -> Multiport Switch1/4
  Constant6/1 -> Multiport Switch1/3
  Bus Selector/4 -> Multiport Switch1/1  "<Charging_State>"
  Multiport Switch1/1 -> Byte Pack1/4

== system Controller_HIL/CAN_Tx/TX_Complete_HIL ==
  Data_0x501 : Inport
  Length_0x501 : Inport  Port=2
  Data_0x502 : Inport  Port=3
  Length_0x502 : Inport  Port=4
  FCAN_Send_ID_0x501 : mbd_s32k1xx_ec_toolbox/Communication Blocks/CAN Blocks/FCAN_Send  Priority=2  can_instance=0  can_mode=Non-blocking  can_timeout_ms=0  can_mb_idx=18  can_mb_init=Once  show_id_input=off  can_extended_id=off  can_is_remote=off  can_id=501  show_adv_opts=on  can_fd_enable=off  can_enable_brs=off  can_fd_padding=0
  FCAN_Send_ID_0x502 : mbd_s32k1xx_ec_toolbox/Communication Blocks/CAN Blocks/FCAN_Send  Priority=2  can_instance=0  can_mode=Non-blocking  can_timeout_ms=0  can_mb_idx=19  can_mb_init=Once  show_id_input=off  can_extended_id=off  can_is_remote=off  can_id=502  show_adv_opts=on  can_fd_enable=off  can_enable_brs=off  can_fd_padding=0
  wires:
  Length_0x502/1 -> FCAN_Send_ID_0x502/2
  Data_0x502/1 -> FCAN_Send_ID_0x502/1
  Data_0x501/1 -> FCAN_Send_ID_0x501/1
  Length_0x501/1 -> FCAN_Send_ID_0x501/2

== system Controller_HIL/CAN_Tx/Tx_Complete ==
  Data_0x201 : Inport
  Length_0x201 : Inport  Port=2
  Data_0x202 : Inport  Port=3
  Length_0x202 : Inport  Port=4
  FCAN_Send_ID_0x201 : mbd_s32k1xx_ec_toolbox/Communication Blocks/CAN Blocks/FCAN_Send  Priority=2  can_instance=0  can_mode=Non-blocking  can_timeout_ms=0  can_mb_idx=16  can_mb_init=Once  show_id_input=off  can_extended_id=off  can_is_remote=off  can_id=201  show_adv_opts=on  can_fd_enable=off  can_enable_brs=off  can_fd_padding=0
  FCAN_Send_ID_0x202 : mbd_s32k1xx_ec_toolbox/Communication Blocks/CAN Blocks/FCAN_Send  Priority=2  can_instance=0  can_mode=Non-blocking  can_timeout_ms=0  can_mb_idx=17  can_mb_init=Once  show_id_input=off  can_extended_id=off  can_is_remote=off  can_id=202  show_adv_opts=on  can_fd_enable=off  can_enable_brs=off  can_fd_padding=0
  wires:
  Length_0x202/1 -> FCAN_Send_ID_0x202/2
  Data_0x202/1 -> FCAN_Send_ID_0x202/1
  Data_0x201/1 -> FCAN_Send_ID_0x201/1
  Length_0x201/1 -> FCAN_Send_ID_0x201/2

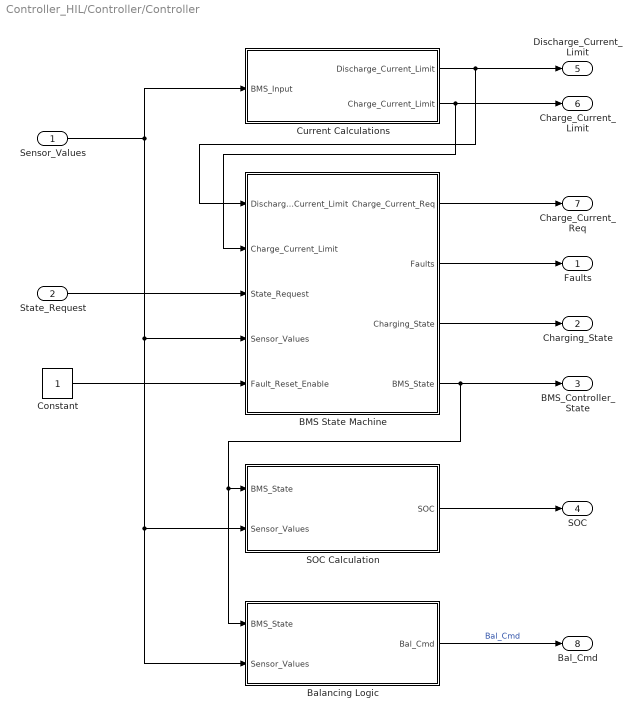
== system Controller_HIL/Controller/Controller ==
  Sensor_Values : Inport  OutDataTypeStr=Bus: Sensor_Values  BusOutputAsStruct=on
  State_Request : Inport  Port=2  OutDataTypeStr=Enum: SRE  PortDimensions=1
  BMS State Machine : Subsystem
  Balancing Logic : Subsystem
  Constant : Constant
  Current Calculations : Subsystem
  SOC Calculation : Subsystem
  Faults : Outport
  Charging_State : Outport  Port=2
  BMS_Controller_State : Outport  Port=3
  SOC : Outport  Port=4
  Discharge_Current_Limit : Outport  Port=5
  Charge_Current_Limit : Outport  Port=6
  Charge_Current_Req : Outport  Port=7
  Bal_Cmd : Outport  Port=8
  wires:
  SOC Calculation/1(SOC) -> SOC/1
  Current Calculations/1(Discharge_Current_Limit) -> BMS State Machine/1(Discharge_Current_Limit), Discharge_Current_Limit/1
  BMS State Machine/2(Faults) -> Faults/1
  BMS State Machine/1(Charge_Current_Req) -> Charge_Current_Req/1
  Sensor_Values/1 -> Balancing Logic/2(Sensor_Values), SOC Calculation/2(Sensor_Values), BMS State Machine/4(Sensor_Values), Current Calculations/1(BMS_Input)
  BMS State Machine/4(BMS_State) -> BMS_Controller_State/1, Balancing Logic/1(BMS_State), SOC Calculation/1(BMS_State)
  Current Calculations/2(Charge_Current_Limit) -> BMS State Machine/2(Charge_Current_Limit), Charge_Current_Limit/1
  Balancing Logic/1(Bal_Cmd) -> Bal_Cmd/1  "Bal_Cmd"
  State_Request/1 -> BMS State Machine/3(State_Request)
  Constant/1 -> BMS State Machine/5(Fault_Reset_Enable)
  BMS State Machine/3(Charging_State) -> Charging_State/1

== system Controller_HIL/CAN Rx/RX_FIFO_Complete_Event/Action_Rx_0x401 ==
  Data : Inport
  Action Port : ActionPort  ActionPortLabel=case [ 1025 ]:
  Byte Unpack : etargetslib/Byte Unpack  dimensions={[1] [1]}  datatypes={'single', 'uint32'}  byteAlign=1
      settings: LibrarySourceBlock=embeddedtargetslib/Host Communication/Byte Unpack
  FCAN_Receive_FIFO : mbd_s32k1xx_ec_toolbox/Communication Blocks/CAN Blocks/FCAN_Receive  can_instance=0  can_mode=Non-blocking  can_timeout_ms=0  can_mb_idx=0  can_mb_init=Once  show_id_input=off  can_extended_id=off  can_is_remote=off  can_id=0x7FF  can_msg_mask=0  show_adv_opts=on  can_use_rxfifo=on  can_fd_enable=off
  Outport : Outport
  Outport1 : Outport  Port=2
  wires:
  Data/1 -> Byte Unpack/1
  Byte Unpack/1 -> Outport/1
  Byte Unpack/2 -> Outport1/1

== system Controller_HIL/CAN Rx/RX_FIFO_Complete_Event/Action_Rx_0x402 ==
  Data : Inport
  Action Port : ActionPort  ActionPortLabel=case [ 1026 ]:
  Byte Unpack : etargetslib/Byte Unpack  dimensions={[1] [1]}  datatypes={'single', 'single'}  byteAlign=1
      settings: LibrarySourceBlock=embeddedtargetslib/Host Communication/Byte Unpack
  FCAN_Receive_FIFO : mbd_s32k1xx_ec_toolbox/Communication Blocks/CAN Blocks/FCAN_Receive  can_instance=0  can_mode=Non-blocking  can_timeout_ms=0  can_mb_idx=0  can_mb_init=Once  show_id_input=off  can_extended_id=off  can_is_remote=off  can_id=0x7FF  can_msg_mask=0  show_adv_opts=on  can_use_rxfifo=on  can_fd_enable=off
  Outport : Outport
  Outport1 : Outport  Port=2
  wires:
  Data/1 -> Byte Unpack/1
  Byte Unpack/1 -> Outport/1
  Byte Unpack/2 -> Outport1/1

== system Controller_HIL/CAN Rx/RX_FIFO_Complete_Event/Action_Rx_0x403 ==
  Data : Inport
  Action Port : ActionPort  ActionPortLabel=case [ 1027 ]:
  Byte Unpack : etargetslib/Byte Unpack  dimensions={[1] [1]}  datatypes={'single', 'single'}  byteAlign=1
      settings: LibrarySourceBlock=embeddedtargetslib/Host Communication/Byte Unpack
  FCAN_Receive_FIFO : mbd_s32k1xx_ec_toolbox/Communication Blocks/CAN Blocks/FCAN_Receive  can_instance=0  can_mode=Non-blocking  can_timeout_ms=0  can_mb_idx=0  can_mb_init=Once  show_id_input=off  can_extended_id=off  can_is_remote=off  can_id=0x7FF  can_msg_mask=0  show_adv_opts=on  can_use_rxfifo=on  can_fd_enable=off
  Outport : Outport
  Outport1 : Outport  Port=2
  wires:
  Data/1 -> Byte Unpack/1
  Byte Unpack/2 -> Outport1/1
  Byte Unpack/1 -> Outport/1

== system Controller_HIL/CAN Rx/RX_FIFO_Complete_Event/Action_Rx_0x404 ==
  Data : Inport
  Action Port : ActionPort  ActionPortLabel=case [ 1028 ]:
  Byte Unpack : etargetslib/Byte Unpack  dimensions={[1] [1]}  datatypes={'single', 'single'}  byteAlign=1
      settings: LibrarySourceBlock=embeddedtargetslib/Host Communication/Byte Unpack
  FCAN_Receive_FIFO : mbd_s32k1xx_ec_toolbox/Communication Blocks/CAN Blocks/FCAN_Receive  can_instance=0  can_mode=Non-blocking  can_timeout_ms=0  can_mb_idx=0  can_mb_init=Once  show_id_input=off  can_extended_id=off  can_is_remote=off  can_id=0x7FF  can_msg_mask=0  show_adv_opts=on  can_use_rxfifo=on  can_fd_enable=off
  Outport : Outport
  Outport1 : Outport  Port=2
  wires:
  Byte Unpack/1 -> Outport/1
  Byte Unpack/2 -> Outport1/1
  Data/1 -> Byte Unpack/1

== system Controller_HIL/CAN Rx/RX_FIFO_Complete_Event/Action_Rx_0x405 ==
  Data : Inport
  Action Port : ActionPort  ActionPortLabel=case [ 1029 ]:
  Byte Unpack : etargetslib/Byte Unpack  dimensions={[1] [1]}  datatypes={'single', 'single'}  byteAlign=1
      settings: LibrarySourceBlock=embeddedtargetslib/Host Communication/Byte Unpack
  FCAN_Receive_FIFO : mbd_s32k1xx_ec_toolbox/Communication Blocks/CAN Blocks/FCAN_Receive  can_instance=0  can_mode=Non-blocking  can_timeout_ms=0  can_mb_idx=0  can_mb_init=Once  show_id_input=off  can_extended_id=off  can_is_remote=off  can_id=0x7FF  can_msg_mask=0  show_adv_opts=on  can_use_rxfifo=on  can_fd_enable=off
  Outport : Outport
  Outport1 : Outport  Port=2
  wires:
  Data/1 -> Byte Unpack/1
  Byte Unpack/1 -> Outport/1
  Byte Unpack/2 -> Outport1/1

== system Controller_HIL/CAN Rx/RX_FIFO_Complete_Event/Action_Rx_0x406 ==
  Data : Inport
  Action Port : ActionPort  ActionPortLabel=case [ 1030 ]:
  Byte Unpack : etargetslib/Byte Unpack  dimensions={[1] [1]}  datatypes={'single', 'single'}  byteAlign=1
      settings: LibrarySourceBlock=embeddedtargetslib/Host Communication/Byte Unpack
  FCAN_Receive_FIFO : mbd_s32k1xx_ec_toolbox/Communication Blocks/CAN Blocks/FCAN_Receive  can_instance=0  can_mode=Non-blocking  can_timeout_ms=0  can_mb_idx=0  can_mb_init=Once  show_id_input=off  can_extended_id=off  can_is_remote=off  can_id=0x7FF  can_msg_mask=0  show_adv_opts=on  can_use_rxfifo=on  can_fd_enable=off
  Outport : Outport
  Outport1 : Outport  Port=2
  wires:
  Data/1 -> Byte Unpack/1
  Byte Unpack/2 -> Outport1/1
  Byte Unpack/1 -> Outport/1

== system Controller_HIL/CAN Rx/RX_FIFO_Complete_Event/Action_Rx_0x407 ==
  Data : Inport
  Action Port : ActionPort  ActionPortLabel=case [ 1031 ]:
  Byte Unpack : etargetslib/Byte Unpack  dimensions={[1] [1]}  datatypes={'single', 'single'}  byteAlign=1
      settings: LibrarySourceBlock=embeddedtargetslib/Host Communication/Byte Unpack
  FCAN_Receive_FIFO : mbd_s32k1xx_ec_toolbox/Communication Blocks/CAN Blocks/FCAN_Receive  can_instance=0  can_mode=Non-blocking  can_timeout_ms=0  can_mb_idx=0  can_mb_init=Once  show_id_input=off  can_extended_id=off  can_is_remote=off  can_id=0x7FF  can_msg_mask=0  show_adv_opts=on  can_use_rxfifo=on  can_fd_enable=off
  Outport : Outport
  Outport1 : Outport  Port=2
  wires:
  Byte Unpack/1 -> Outport/1
  Byte Unpack/2 -> Outport1/1
  Data/1 -> Byte Unpack/1

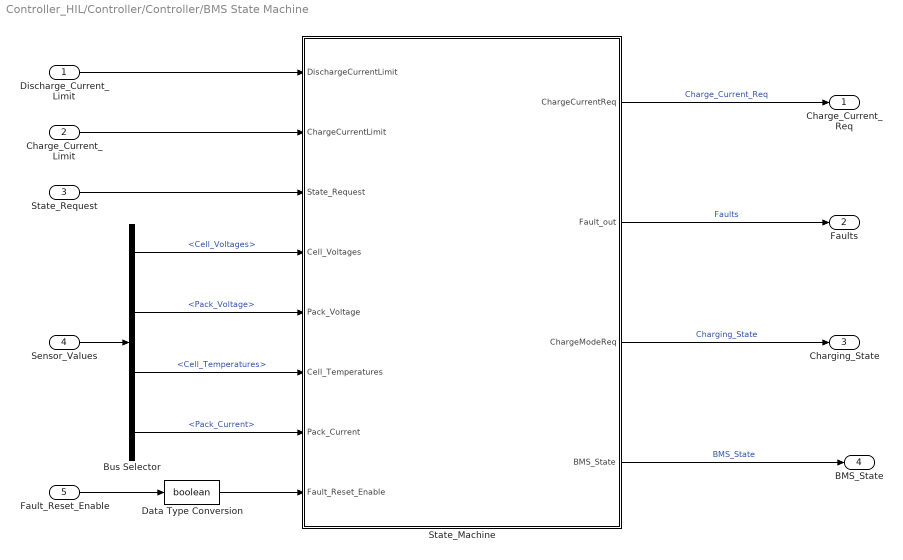
== system Controller_HIL/Controller/Controller/BMS State Machine ==
  Discharge_Current_Limit : Inport
  Charge_Current_Limit : Inport  Port=2
  State_Request : Inport  Port=3  OutDataTypeStr=Enum: SRE
  Sensor_Values : Inport  Port=4
  Fault_Reset_Enable : Inport  Port=5
  Bus Selector : BusSelector  OutputSignals=Cell_Voltages,Pack_Voltage,Cell_Temperatures,Pack_Current
  Data Type Conversion : DataTypeConversion  OutDataTypeStr=boolean  SaturateOnIntegerOverflow=off  RndMeth=Floor
  State_Machine : Stateflow chart  TreatAsAtomicUnit=on  VariantControl=(default)
  Charge_Current_Req : Outport  OutMin=-100  OutMax=100  OutDataTypeStr=single  VectorParamsAs1DForOutWhenUnconnected=off
  Faults : Outport  Port=2  OutDataTypeStr=Bus: Faults  VectorParamsAs1DForOutWhenUnconnected=off  BusOutputAsStruct=on
  Charging_State : Outport  Port=3
  BMS_State : Outport  Port=4  OutDataTypeStr=Enum: BMS_Controller_State  VectorParamsAs1DForOutWhenUnconnected=off
  wires:
  State_Machine/2(Fault_out) -> Faults/1  "Faults"
  Bus Selector/1 -> State_Machine/4(Cell_Voltages)  "<Cell_Voltages>"
  State_Machine/1(ChargeCurrentReq) -> Charge_Current_Req/1  "Charge_Current_Req"
  State_Request/1 -> State_Machine/3(State_Request)
  Discharge_Current_Limit/1 -> State_Machine/1(DischargeCurrentLimit)
  Charge_Current_Limit/1 -> State_Machine/2(ChargeCurrentLimit)
  Bus Selector/3 -> State_Machine/6(Cell_Temperatures)  "<Cell_Temperatures>"
  Bus Selector/2 -> State_Machine/5(Pack_Voltage)  "<Pack_Voltage>"
  Bus Selector/4 -> State_Machine/7(Pack_Current)  "<Pack_Current>"
  Sensor_Values/1 -> Bus Selector/1
  Fault_Reset_Enable/1 -> Data Type Conversion/1
  Data Type Conversion/1 -> State_Machine/8(Fault_Reset_Enable)
  State_Machine/3(ChargeModeReq) -> Charging_State/1  "Charging_State"
  State_Machine/4(BMS_State) -> BMS_State/1  "BMS_State"

== system Controller_HIL/Controller/Controller/Balancing Logic ==
  BMS_State : Inport  OutDataTypeStr=Enum: BMS_Controller_State  PortDimensions=1
  Sensor_Values : Inport  Port=2
  Balancing : Stateflow chart  TreatAsAtomicUnit=on  VariantControl=(default)
  Bus Selector1 : BusSelector  OutputSignals=Cell_Voltages
  Bal_Cmd : Outport  OutDataTypeStr=boolean  PortDimensions=[1,NumModules*Ns_Module]  VectorParamsAs1DForOutWhenUnconnected=off
  wires:
  Balancing/1(Bal_Cmd) -> Bal_Cmd/1  "Bal_Cmd"
  Bus Selector1/1 -> Balancing/2(CellVoltages)  "<Cell_Voltages>"
  Sensor_Values/1 -> Bus Selector1/1
  BMS_State/1 -> Balancing/1(BMS_State)

== system Controller_HIL/Controller/Controller/Current Calculations ==
  BMS_Input : Inport
  Bus Selector : BusSelector  OutputSignals=Cell_Voltages,Cell_Temperatures
  Charge_Current_Limit_Calc : Subsystem
  Discharge_Current_Limit_Calc : Subsystem
  MinMax : MinMax
  MinMax1 : MinMax
  MinMax2 : MinMax  Function=max
  MinMax4 : MinMax  Function=max
  Discharge_Current_Limit : Outport
  Charge_Current_Limit : Outport  Port=2
  wires:
  MinMax/1 -> Discharge_Current_Limit_Calc/1(MinCellVolt)  "Min_Cell_Volt"
  MinMax4/1 -> Discharge_Current_Limit_Calc/3(MaxCellTemp), Charge_Current_Limit_Calc/3(MaxCellTemp)  "Max_Cell_Temp"
  MinMax1/1 -> Discharge_Current_Limit_Calc/2(MinCellTemp), Charge_Current_Limit_Calc/2(MinCellTemp)  "Min_Cell_Temp"
  MinMax2/1 -> Charge_Current_Limit_Calc/1(MaxCellVolt)  "Max_Cell_Volt"
  Discharge_Current_Limit_Calc/1(Discharge_Current_Limit) -> Discharge_Current_Limit/1  "Discharge_Current_Limit"
  Charge_Current_Limit_Calc/1(Charge_Current_Limit) -> Charge_Current_Limit/1  "Charge_Current_Limit"
  Bus Selector/1 -> MinMax/1, MinMax2/1  "<Cell_Voltages>"
  Bus Selector/2 -> MinMax4/1, MinMax1/1  "<Cell_Temperatures>"
  BMS_Input/1 -> Bus Selector/1

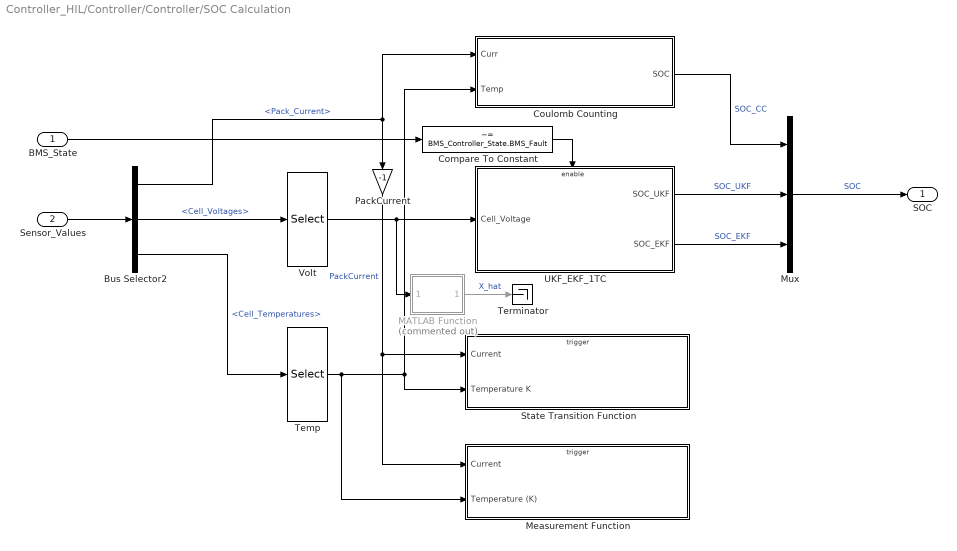
== system Controller_HIL/Controller/Controller/SOC Calculation ==
  BMS_State : Inport  OutDataTypeStr=Enum: BMS_Controller_State
  Sensor_Values : Inport  Port=2
  Bus Selector2 : BusSelector  OutputSignals=Pack_Current,Cell_Voltages,Cell_Temperatures
  Compare To Constant : simulink/Logic and Bit Operations/Compare To Constant  relop=~=  const=BMS_Controller_State.BMS_Fault  OutDataTypeStr=boolean
  Coulomb Counting : Subsystem  VariantControl=SocAlgo==1
  MATLAB Function : MATLAB Function  Commented=on  TreatAsAtomicUnit=on
  Measurement Function : Subsystem  TreatAsAtomicUnit=on
  Mux : Mux  Inputs=3
  PackCurrent : Gain  Gain=-1
  State Transition Function : Subsystem  TreatAsAtomicUnit=on
  Temp : Selector  InputPortWidth=Ns_Module*NumModules  IndexOptions=Index vector (dialog)  Indices=1  OutputSizes=1
  Terminator : Terminator
  UKF_EKF_1TC : Subsystem  VariantControl=CellType==1
  Volt : Selector  InputPortWidth=Ns_Module*NumModules  IndexOptions=Index vector (dialog)  Indices=1  OutputSizes=1
  SOC : Outport  OutDataTypeStr=single  VectorParamsAs1DForOutWhenUnconnected=off
  wires:
  Mux/1 -> SOC/1  "SOC"
  UKF_EKF_1TC/1(SOC_UKF) -> Mux/2  "SOC_UKF"
  BMS_State/1 -> Compare To Constant/1
  Coulomb Counting/1(SOC) -> Mux/1  "SOC_CC"
  Volt/1 -> MATLAB Function/1(meas), UKF_EKF_1TC/1(Cell_Voltage)
  MATLAB Function/1(xhatOut) -> Terminator/1  "X_hat"
  Temp/1 -> Coulomb Counting/2(Temp), State Transition Function/2(Temperature K), Measurement Function/2(Temperature (K))
  Compare To Constant/1 -> UKF_EKF_1TC/Enable
  UKF_EKF_1TC/2(SOC_EKF) -> Mux/3  "SOC_EKF"
  Bus Selector2/1 -> Coulomb Counting/1(Curr), PackCurrent/1  "<Pack_Current>"
  PackCurrent/1 -> State Transition Function/1(Current), Measurement Function/1(Current)  "PackCurrent"
  Bus Selector2/3 -> Temp/1  "<Cell_Temperatures>"
  Bus Selector2/2 -> Volt/1  "<Cell_Voltages>"
  Sensor_Values/1 -> Bus Selector2/1

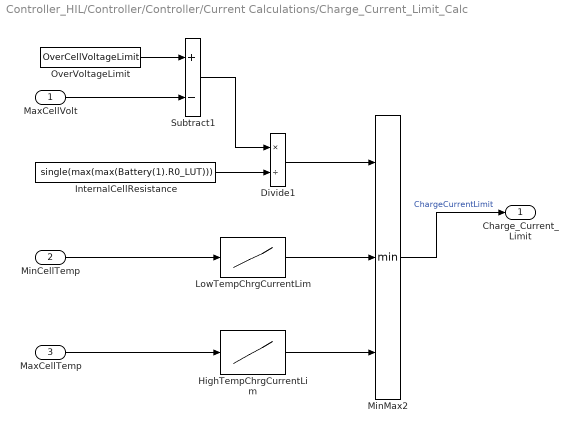
== system Controller_HIL/Controller/Controller/Current Calculations/Charge_Current_Limit_Calc ==
  MaxCellVolt : Inport
  MinCellTemp : Inport  Port=2
  MaxCellTemp : Inport  Port=3
  Divide1 : Product  Inputs=*/
  HighTempChrgCurrentLim : Lookup_n-D  NumberOfTableDimensions=1  BreakpointsForDimension1=273.15+[-30:1:70]  Table=50*(1-tanh(273.15+[-30:1:70]-273.15-50))/2  InternalRulePriority=Speed  RndMeth=Simplest
  InternalCellResistance : Constant  Value=single(max(max(Battery(1).R0_LUT)))  OutDataTypeStr=single  SampleTime=-1
  LowTempChrgCurrentLim : Lookup_n-D  NumberOfTableDimensions=1  BreakpointsForDimension1=273.15+[-30:1:70]  Table=50*(1+tanh(273.15+[-30:1:70]-(273.15)))/2  InternalRulePriority=Speed  RndMeth=Simplest
  MinMax2 : MinMax  Inputs=3
  OverVoltageLimit : Constant  Value=OverCellVoltageLimit  OutDataTypeStr=single  SampleTime=-1
  Subtract1 : Sum  Inputs=+-
  Charge_Current_Limit : Outport  VectorParamsAs1DForOutWhenUnconnected=off
  wires:
  OverVoltageLimit/1 -> Subtract1/1
  MinMax2/1 -> Charge_Current_Limit/1  "ChargeCurrentLimit"
  MaxCellVolt/1 -> Subtract1/2
  Subtract1/1 -> Divide1/1
  Divide1/1 -> MinMax2/1
  InternalCellResistance/1 -> Divide1/2
  MinCellTemp/1 -> LowTempChrgCurrentLim/1
  MaxCellTemp/1 -> HighTempChrgCurrentLim/1
  HighTempChrgCurrentLim/1 -> MinMax2/3
  LowTempChrgCurrentLim/1 -> MinMax2/2

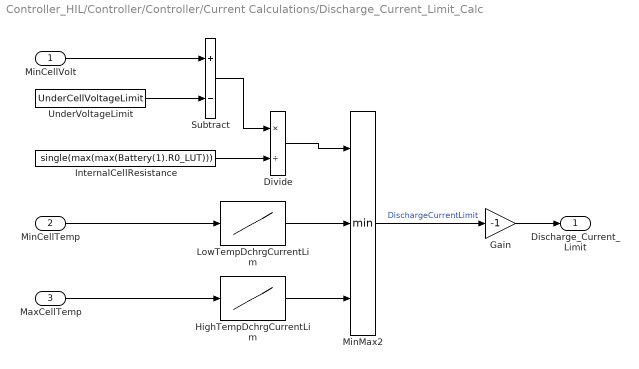
== system Controller_HIL/Controller/Controller/Current Calculations/Discharge_Current_Limit_Calc ==
  MinCellVolt : Inport
  MinCellTemp : Inport  Port=2
  MaxCellTemp : Inport  Port=3
  Divide : Product  Inputs=*/
  Gain : Gain  Gain=-1
  HighTempDchrgCurrentLim : Lookup_n-D  NumberOfTableDimensions=1  BreakpointsForDimension1=273.15+[-30:1:70]  Table=100*(1-tanh(273.15+[-30:1:70]-273.15-50))/2  InternalRulePriority=Speed  RndMeth=Simplest
  InternalCellResistance : Constant  Value=single(max(max(Battery(1).R0_LUT)))  OutDataTypeStr=single  SampleTime=-1
  LowTempDchrgCurrentLim : Lookup_n-D  NumberOfTableDimensions=1  BreakpointsForDimension1=273.15+[-30:1:70]  Table=100*(1+tanh(273.15+[-30:1:70]-(273.15)))/2  InternalRulePriority=Speed  RndMeth=Simplest
  MinMax2 : MinMax  Inputs=3
  Subtract : Sum  Inputs=+-
  UnderVoltageLimit : Constant  Value=UnderCellVoltageLimit  OutDataTypeStr=single  SampleTime=-1
  Discharge_Current_Limit : Outport  VectorParamsAs1DForOutWhenUnconnected=off
  wires:
  MinMax2/1 -> Gain/1  "DischargeCurrentLimit"
  Divide/1 -> MinMax2/1
  MinCellVolt/1 -> Subtract/1
  InternalCellResistance/1 -> Divide/2
  Subtract/1 -> Divide/1
  UnderVoltageLimit/1 -> Subtract/2
  Gain/1 -> Discharge_Current_Limit/1
  MaxCellTemp/1 -> HighTempDchrgCurrentLim/1
  MinCellTemp/1 -> LowTempDchrgCurrentLim/1
  HighTempDchrgCurrentLim/1 -> MinMax2/3
  LowTempDchrgCurrentLim/1 -> MinMax2/2

== system Controller_HIL/Controller/Controller/SOC Calculation/Coulomb Counting ==
  Curr : Inport
  Temp : Inport  Port=2
  1-D Lookup Table : Lookup_n-D  NumberOfTableDimensions=1  BreakpointsForDimension1=single(Battery(1).Temperature_LUT)  Table=single(Battery(1).Capacity_LUT)  InternalRulePriority=Speed  RndMeth=Simplest
  Discrete-Time Integrator : DiscreteIntegrator  InitialCondition=single(SOCInit+0.05)  SampleTime=-1  LimitOutput=on  UpperSaturationLimit=1  LowerSaturationLimit=0  ICPrevOutput=DiscIntNeverNeededParam  ICPrevScaledInput=DiscIntNeverNeededParam
  Divide : Product  Inputs=*/
  Gain : Gain  Gain=single(1/3600)
  SOC : Outport  VectorParamsAs1DForOutWhenUnconnected=off
  wires:
  Discrete-Time Integrator/1 -> SOC/1
  Curr/1 -> Gain/1
  Gain/1 -> Divide/1
  Divide/1 -> Discrete-Time Integrator/1
  1-D Lookup Table/1 -> Divide/2  "Capacity"
  Temp/1 -> 1-D Lookup Table/1
